simulink model "mpc_uncon"  (R2019b)
settings: Solver=VariableStepAuto  StartTime=0.0  StopTime=time_end  RelTol=1e-3
values from neighbouring files (symbols this model uses):
  h_01 = 10.17    [script_mpc_uncon.m]
  h_02 = 10.53    [script_mpc_uncon.m]
  ue = [ue1; ue2]    [script_mpc_uncon.m]
  xe = [xe1; xe2]    [script_mpc_uncon.m]
undefined symbols (not defined in the file or in its folder): A, B, C, F, G, K
settings Model: Creator=NicSch02  LastModifiedBy=NicSch02

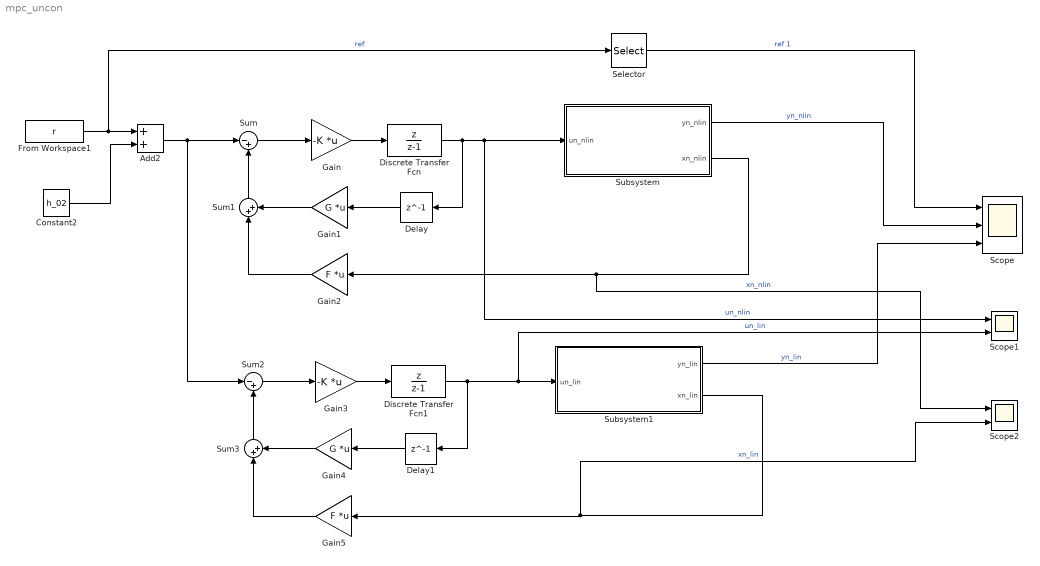
== system mpc_uncon ==
  Add2 : Sum
  Constant2 : Constant  Value=h_02
  Delay : Delay  DelayLength=1
  Delay1 : Delay  DelayLength=1
  Discrete Transfer Fcn : DiscreteTransferFcn  Numerator=[1 0]  Denominator=[1 -1]  SampleTime=0.5
  Discrete Transfer Fcn1 : DiscreteTransferFcn  Numerator=[1 0]  Denominator=[1 -1]  SampleTime=0.5
  From Workspace1 : FromWorkspace  VariableName=r  SampleTime=0
  Gain : Gain  Gain=-K  Multiplication=Matrix(K*u)
  Gain1 : Gain  Gain=G  Multiplication=Matrix(K*u)
  Gain2 : Gain  Gain=F  Multiplication=Matrix(K*u)
  Gain3 : Gain  Gain=-K  Multiplication=Matrix(K*u)
  Gain4 : Gain  Gain=G  Multiplication=Matrix(K*u)
  Gain5 : Gain  Gain=F  Multiplication=Matrix(K*u)
  Scope : Scope  NumInputPorts=3
  Scope1 : Scope  NumInputPorts=2
  Scope2 : Scope  NumInputPorts=2
  Selector : Selector  InputPortWidth=Np  IndexOptions=Index vector (dialog)  Indices=[1]  OutputSizes=1
  Subsystem : Subsystem
  Subsystem1 : Subsystem
  Sum : Sum  Inputs=|-+
  Sum1 : Sum  Inputs=|++
  Sum2 : Sum  Inputs=|-+
  Sum3 : Sum  Inputs=|++
  wires:
  Sum/1 -> Gain/1
  Gain/1 -> Discrete Transfer Fcn/1
  Discrete Transfer Fcn/1 -> Scope1/1, Subsystem/1(un_nlin), Delay/1  "un_nlin"
  Delay/1 -> Gain1/1
  Gain1/1 -> Sum1/2
  Sum1/1 -> Sum/2
  Gain2/1 -> Sum1/1
  Subsystem/1(yn_nlin) -> Scope/2  "yn_nlin"
  Discrete Transfer Fcn1/1 -> Scope1/2, Subsystem1/1(un_lin), Delay1/1  "un_lin"
  Gain4/1 -> Sum3/2
  Gain3/1 -> Discrete Transfer Fcn1/1
  Delay1/1 -> Gain4/1
  Sum3/1 -> Sum2/2
  Sum2/1 -> Gain3/1
  Gain5/1 -> Sum3/1
  Subsystem/2(xn_nlin) -> Scope2/1, Gain2/1  "xn_nlin"
  Subsystem1/2(xn_lin) -> Scope2/2, Gain5/1  "xn_lin"
  Selector/1 -> Scope/1  "ref 1"
  Add2/1 -> Sum2/1, Sum/1
  From Workspace1/1 -> Selector/1, Add2/1  "ref"
  Constant2/1 -> Add2/2
  Subsystem1/1(yn_lin) -> Scope/3  "yn_lin"

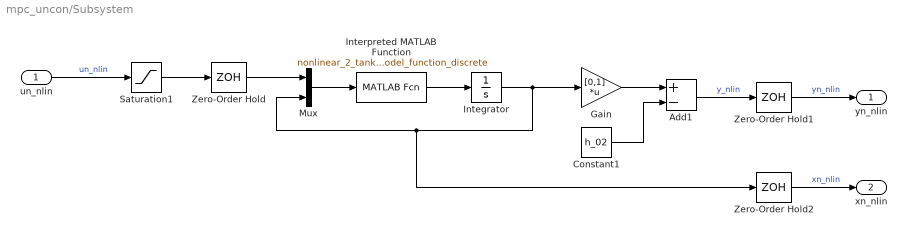
== system mpc_uncon/Subsystem ==
  un_nlin : Inport
  Add1 : Sum  Inputs=+-
  Constant1 : Constant  Value=h_02
  Gain : Gain  Gain=[0,1]  Multiplication=Matrix(K*u)
  Integrator : Integrator  InitialCondition=[h_01;h_02]
  Interpreted MATLAB Function : MATLABFcn  MATLABFcn=nonlinear_2_tank_model_function_discrete
  Mux : Mux  Inputs=2
  Saturation1 : Saturate  UpperLimit=5  LowerLimit=0
  Zero-Order Hold : ZeroOrderHold  SampleTime=0.5
  Zero-Order Hold1 : ZeroOrderHold  SampleTime=0.5
  Zero-Order Hold2 : ZeroOrderHold  SampleTime=0.5
  yn_nlin : Outport
  xn_nlin : Outport  Port=2
  wires:
  Integrator/1 -> Zero-Order Hold2/1, Mux/2, Gain/1
  Constant1/1 -> Add1/2
  Interpreted MATLAB Function/1 -> Integrator/1
  Gain/1 -> Add1/1
  Mux/1 -> Interpreted MATLAB Function/1
  un_nlin/1 -> Saturation1/1  "un_nlin"
  Zero-Order Hold/1 -> Mux/1
  Add1/1 -> Zero-Order Hold1/1  "y_nlin"
  Zero-Order Hold1/1 -> yn_nlin/1  "yn_nlin"
  Saturation1/1 -> Zero-Order Hold/1
  Zero-Order Hold2/1 -> xn_nlin/1  "xn_nlin"

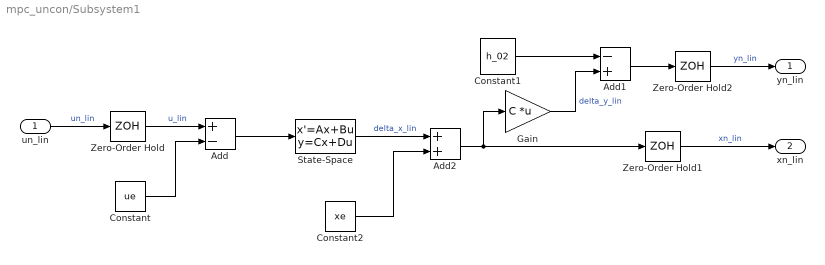
== system mpc_uncon/Subsystem1 ==
  un_lin : Inport
  Add : Sum  Inputs=+-
  Add1 : Sum  Inputs=-+
  Add2 : Sum
  Constant : Constant  Value=ue
  Constant1 : Constant  Value=h_02
  Constant2 : Constant  Value=xe
  Gain : Gain  Gain=C  Multiplication=Matrix(K*u)
  State-Space : StateSpace  A=A  B=B  C=[[1,0];[0,1]]  D=[[0,0];[0,0]]  InitialCondition=[h_01;h_02] - xe
  Zero-Order Hold : ZeroOrderHold  SampleTime=-1
  Zero-Order Hold1 : ZeroOrderHold  SampleTime=-1
  Zero-Order Hold2 : ZeroOrderHold  SampleTime=-1
  yn_lin : Outport
  xn_lin : Outport  Port=2
  wires:
  un_lin/1 -> Zero-Order Hold/1  "un_lin"
  Zero-Order Hold1/1 -> xn_lin/1  "xn_lin"
  Zero-Order Hold2/1 -> yn_lin/1  "yn_lin"
  Add1/1 -> Zero-Order Hold2/1
  Constant1/1 -> Add1/1
  Gain/1 -> Add1/2  "delta_y_lin"
  Zero-Order Hold/1 -> Add/1  "u_lin"
  Constant/1 -> Add/2
  Add/1 -> State-Space/1
  State-Space/1 -> Add2/1  "delta_x_lin"
  Add2/1 -> Gain/1, Zero-Order Hold1/1
  Constant2/1 -> Add2/2
